simulink model "sensor_subsystem"  (R2023b)
settings: Solver=VariableStepAuto  StartTime=0.0  StopTime=10.0  RelTol=1e-3
settings Model: Creator=tiwan  LastModifiedBy=tiwan

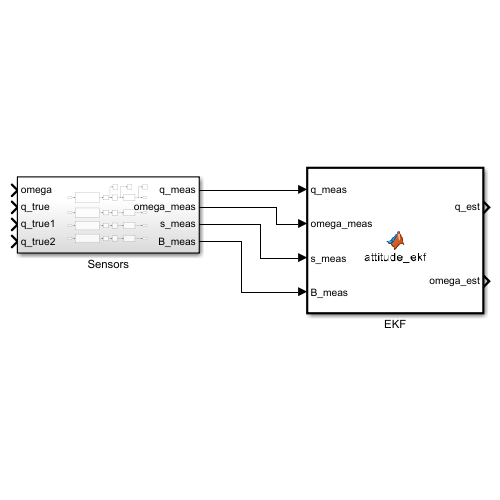
[thumbnail: Simulink's stored preview of the top-level diagram]
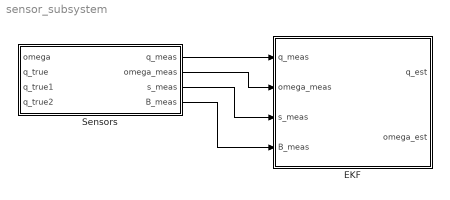
== system sensor_subsystem ==
  EKF : MATLAB Function  TreatAsAtomicUnit=on
  Sensors : Subsystem
  wires:
  Sensors/1(q_meas) -> EKF/1(q_meas)
  Sensors/2(omega_meas) -> EKF/2(omega_meas)
  Sensors/3(s_meas) -> EKF/3(s_meas)
  Sensors/4(B_meas) -> EKF/4(B_meas)

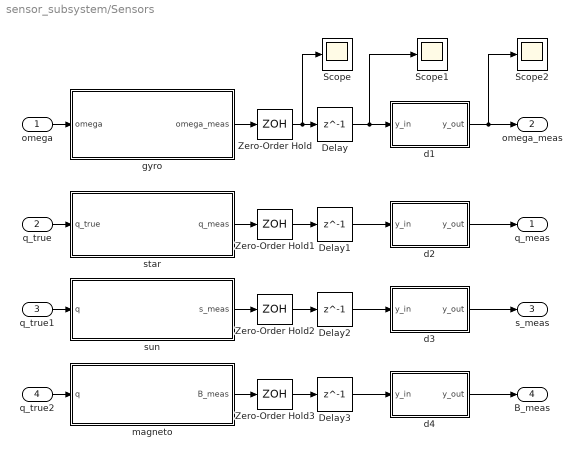
== system sensor_subsystem/Sensors ==
  omega : Inport
  q_true : Inport  Port=2
  q_true1 : Inport  Port=3
  q_true2 : Inport  Port=4
  Delay{,1..3} (4 alike) : Delay  DelayLength=1  InitialCondition=0  SampleTime=0.05
  Scope : Scope
  Scope1 : Scope
  Scope2 : Scope
  Zero-Order Hold : ZeroOrderHold  SampleTime=0.1
  Zero-Order Hold1 : ZeroOrderHold  SampleTime=-1
  Zero-Order Hold2 : ZeroOrderHold  SampleTime=-1
  Zero-Order Hold3 : ZeroOrderHold  SampleTime=-1
  d1 : MATLAB Function  TreatAsAtomicUnit=on
  d2 : MATLAB Function  TreatAsAtomicUnit=on
  d3 : MATLAB Function  TreatAsAtomicUnit=on
  d4 : MATLAB Function  TreatAsAtomicUnit=on
  gyro : MATLAB Function  TreatAsAtomicUnit=on
  magneto : MATLAB Function  TreatAsAtomicUnit=on
  star : MATLAB Function  TreatAsAtomicUnit=on
  sun : MATLAB Function  TreatAsAtomicUnit=on
  q_meas : Outport
  omega_meas : Outport  Port=2
  s_meas : Outport  Port=3
  B_meas : Outport  Port=4
  wires:
  omega/1 -> gyro/1(omega)
  q_true/1 -> star/1(q_true)
  star/1(q_meas) -> Zero-Order Hold1/1
  gyro/1(omega_meas) -> Zero-Order Hold/1
  Zero-Order Hold/1 -> Scope/1, Delay/1
  Zero-Order Hold1/1 -> Delay1/1
  Delay/1 -> Scope1/1, d1/1(y_in)
  Delay1/1 -> d2/1(y_in)
  d2/1(y_out) -> q_meas/1
  q_true1/1 -> sun/1(q)
  q_true2/1 -> magneto/1(q)
  magneto/1(B_meas) -> Zero-Order Hold3/1
  sun/1(s_meas) -> Zero-Order Hold2/1
  Zero-Order Hold2/1 -> Delay2/1
  Zero-Order Hold3/1 -> Delay3/1
  Delay2/1 -> d3/1(y_in)
  Delay3/1 -> d4/1(y_in)
  d3/1(y_out) -> s_meas/1
  d4/1(y_out) -> B_meas/1
  d1/1(y_out) -> Scope2/1, omega_meas/1

== matlab function sensor_subsystem/Sensors/gyro ==
  settings: updateMethod=DISCRETE
  data: omega input; omega_meas output
function omega_meas = gyro_sensor(omega)
% Simple gyroscope with bias and Gaussian noise
bias = [0.0005; -0.0003; 0.0004];     % Constant bias (rad/s)
noise_std = 0.001;                    % Noise std dev (rad/s)

omega_meas = omega + bias + noise_std * randn(3,1);
end

== matlab function sensor_subsystem/Sensors/star ==
  settings: updateMethod=DISCRETE
  data: q_true input; q_meas output
function q_meas = star_tracker(q_true)
% Star tracker with small attitude noise
noise_std = 0.002;

q_meas = q_true + noise_std * randn(4,1);
q_meas = q_meas / norm(q_meas);  % Normalize to unit quaternion
end

== matlab function sensor_subsystem/Sensors/d1 ==
  data: y_in input; y_out output
function y_out = dropout(y_in)
% Simulate dropout with 2% chance
if rand < 0.02
    y_out = zeros(size(y_in));  % Lost reading
else
    y_out = y_in;
end
end

== matlab function sensor_subsystem/Sensors/d2 ==
  data: y_in input; y_out output
function y_out = dropout(y_in)
% Simulate dropout with 2% chance
if rand < 0.02
    y_out = zeros(size(y_in));  % Lost reading
else
    y_out = y_in;
end
end

== matlab function sensor_subsystem/Sensors/sun ==
  settings: updateMethod=DISCRETE
  data: q input; s_meas output
function s_meas = sun_sensor(q)
% Constants
s_inertial = [-1; 0; 0];           % Sun vector in inertial frame (unit vector)
noise_std = 0.01;                  % Sun sensor noise

% Convert quaternion to rotation matrix
q0 = q(1); qv = q(2:4);
q_cross = [    0   -qv(3)  qv(2);
            qv(3)     0   -qv(1);
           -qv(2)  qv(1)     0 ];
R = (q0^2 - qv' * qv) * eye(3) + 2 * (qv * qv') - 2 * q0 * q_cross;

% Transform Sun vector to body frame
s_body = R * s_inertial;

% Add noise
s_meas = s_body + noise_std * randn(3,1);
end

== matlab function sensor_subsystem/Sensors/magneto ==
  settings: updateMethod=DISCRETE
  data: q input; B_meas output
function B_meas = magnetometer(q)
% Constants
B_inertial = [0.2; -0.3; 0.4];     % Earth's magnetic field in inertial frame (μT)
noise_std = 0.01;                  % Magnetometer noise

% Convert quaternion to rotation matrix
q0 = q(1); qv = q(2:4);
q_cross = [    0   -qv(3)  qv(2);
            qv(3)     0   -qv(1);
           -qv(2)  qv(1)     0 ];
R = (q0^2 - qv' * qv) * eye(3) + 2 * (qv * qv') - 2 * q0 * q_cross;

% Transform magnetic field vector to body frame
B_body = R * B_inertial;

% Add noise
B_meas = B_body + noise_std * randn(3,1);
end

== matlab function sensor_subsystem/EKF ==
  data: q_meas input; q_est output; omega_meas input; s_meas input; B_meas input; omega_est output
function [q_est, omega_est] = attitude_ekf(q_meas, omega_meas, s_meas, B_meas)

% ======= Input Guards =======
if isempty(q_meas) || norm(q_meas) == 0 || any(isnan(q_meas))
    q_meas = [1; 0; 0; 0];  % fallback to identity quaternion
end

if isempty(omega_meas) || any(isnan(omega_meas))
    omega_meas = [0; 0; 0];
end

% ======= Persistent Variables =======
persistent x P
dt = 0.01;

if isempty(x)
    x = [q_meas; omega_meas];     % Initial state
    P = 1e-2 * eye(7);             % Initial covariance
end

% ======= Prediction Step =======
q = x(1:4);
omega = x(5:7);

% Quaternion derivative using Omega matrix
Omega = [0, -omega';
         omega, -skew(omega)];

q_dot = 0.5 * Omega * q;
q_pred = q + dt * q_dot;

% Normalize prediction
if norm(q_pred) == 0 || any(isnan(q_pred))
    q_pred = [1; 0; 0; 0];
else
    q_pred = q_pred / norm(q_pred);
end

omega_pred = omega;

% Jacobians (simplified)
F = eye(7);
Q = 1e-4 * eye(7);

x_pred = [q_pred; omega_pred];
P = F * P * F' + Q;

% ======= Measurement Update =======
H = eye(7);                 % Direct observation
R = 1e-3 * eye(7);           % Measurement noise

z = [q_meas; omega_meas];  % Measurement vector
z_pred = x_pred;           % Predicted measurement

% Kalman Gain
K = P * H' / (H * P * H' + R);

% EKF Update
x = x_pred + K * (z - z_pred);

% Normalize quaternion again
if norm(x(1:4)) == 0 || any(isnan(x(1:4)))
    x(1:4) = [1; 0; 0; 0];
else
    x(1:4) = x(1:4) / norm(x(1:4));
end

P = (eye(7) - K * H) * P;

% ======= Outputs =======
q_est = x(1:4);
omega_est = x(5:7);

end

% ======= Helper Function =======
function S = skew(w)
S = [ 0    -w(3)  w(2);
      w(3)  0    -w(1);
     -w(2)  w(1)  0   ];
end

== matlab function sensor_subsystem/Sensors/d3 ==
  data: y_in input; y_out output
function y_out = dropout(y_in)
% Simulate dropout with 2% chance
if rand < 0.02
    y_out = zeros(size(y_in));  % Lost reading
else
    y_out = y_in;
end
end

== matlab function sensor_subsystem/Sensors/d4 ==
  data: y_in input; y_out output
function y_out = dropout(y_in)
% Simulate dropout with 2% chance
if rand < 0.02
    y_out = zeros(size(y_in));  % Lost reading
else
    y_out = y_in;
end
end
